simulink model "TrajectoryGenerator2DOF_freq"  (R2023b)
settings: Solver=FixedStepDiscrete  StartTime=0.0  StopTime=1.2*1.4  FixedStep=0.002  RelTol=1e-3
undefined symbols (not defined in the file or in its folder): M_z, Smoothers, Ts
(part 1 of 2)
settings Model: Creator=simon  LastModifiedBy=simon

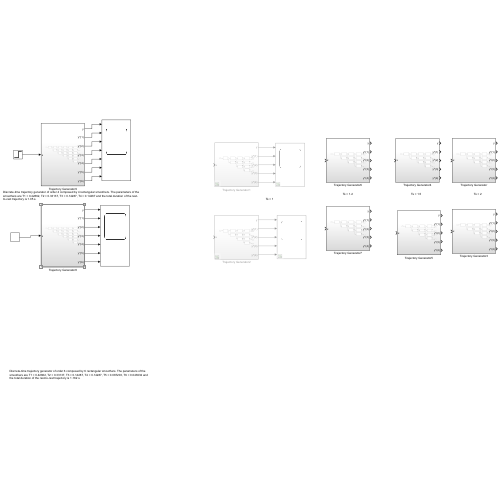
[thumbnail: Simulink's stored preview of the top-level diagram]
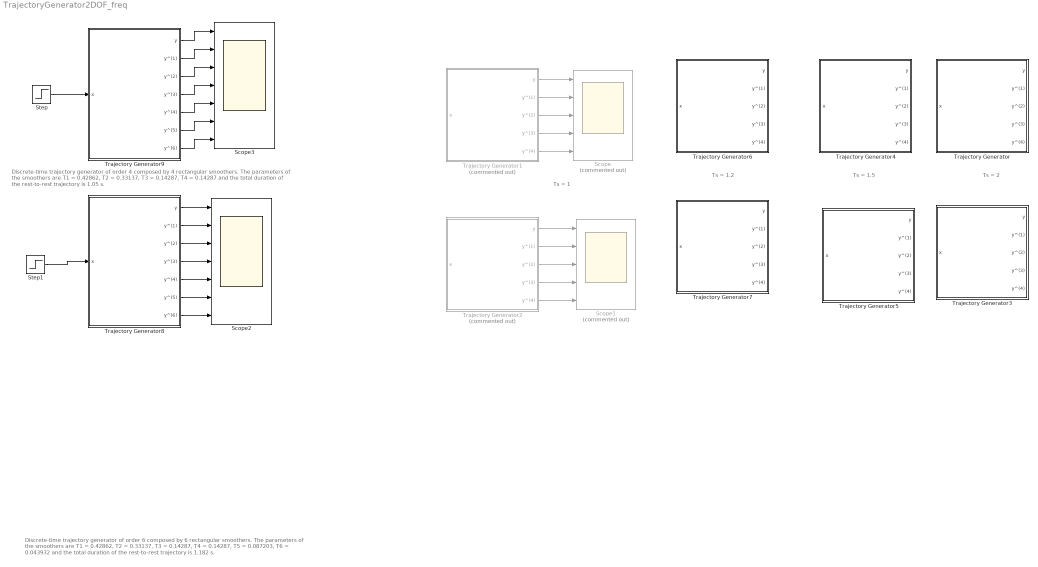
== system TrajectoryGenerator2DOF_freq ==
  note: Ts = 1
  note: Discrete-time trajectory generator of order 4 composed by 4 rectangular smoothers. The parameters of the smoothers are T1 = 0.42862, T2 = 0.33137, T3 = 0.14287, T4 = 0.14287 and the total duration of the rest-to-rest trajectory is 1.05 s.
  note: Ts = 2
  note: Ts = 1.5
  note: Ts = 1.2
  note: Discrete-time trajectory generator of order 6 composed by 6 rectangular smoothers. The parameters of the smoothers are T1 = 0.42862, T2 = 0.33137, T3 = 0.14287, T4 = 0.14287, T5 = 0.087203, T6 = 0.043932 and the total duration of the rest-to-rest trajectory is 1.182 s.
  Scope : Scope  Commented=on  NumInputPorts=5
  Scope1 : Scope  Commented=on  NumInputPorts=5
  Scope2 : Scope  NumInputPorts=7
  Scope3 : Scope  NumInputPorts=7
  Step : Step  Time=0  After=0.5  SampleTime=0.002
  Step1 : Step  Time=0.4*Ts  After=-0.5  SampleTime=0.002
  Trajectory Generator : Subsystem
  Trajectory Generator1 : Subsystem  Commented=on
  Trajectory Generator2 : Subsystem  Commented=on
  Trajectory Generator3 : Subsystem
  Trajectory Generator4 : Subsystem
  Trajectory Generator5 : Subsystem
  Trajectory Generator6 : Subsystem
  Trajectory Generator7 : Subsystem
  Trajectory Generator8 : Subsystem
  Trajectory Generator9 : Subsystem
  wires:
  Step/1 -> Trajectory Generator9/1(x)
  Step1/1 -> Trajectory Generator8/1(x)
  Trajectory Generator8/6(y^(5)) -> Scope2/6
  Trajectory Generator8/4(y^(3)) -> Scope2/4
  Trajectory Generator8/7(y^(6)) -> Scope2/7
  Trajectory Generator8/3(y^(2)) -> Scope2/3
  Trajectory Generator8/5(y^(4)) -> Scope2/5
  Trajectory Generator8/2(y^(1)) -> Scope2/2
  Trajectory Generator8/1(y) -> Scope2/1
  Trajectory Generator1/4(y^(3)) -> Scope/4
  Trajectory Generator1/5(y^(4)) -> Scope/5
  Trajectory Generator1/2(y^(1)) -> Scope/2
  Trajectory Generator1/1(y) -> Scope/1
  Trajectory Generator1/3(y^(2)) -> Scope/3
  Trajectory Generator9/5(y^(4)) -> Scope3/5
  Trajectory Generator9/1(y) -> Scope3/1
  Trajectory Generator9/2(y^(1)) -> Scope3/2
  Trajectory Generator9/4(y^(3)) -> Scope3/4
  Trajectory Generator9/3(y^(2)) -> Scope3/3
  Trajectory Generator9/6(y^(5)) -> Scope3/6
  Trajectory Generator9/7(y^(6)) -> Scope3/7
  Trajectory Generator2/2(y^(1)) -> Scope1/2
  Trajectory Generator2/3(y^(2)) -> Scope1/3
  Trajectory Generator2/4(y^(3)) -> Scope1/4
  Trajectory Generator2/5(y^(4)) -> Scope1/5
  Trajectory Generator2/1(y) -> Scope1/1

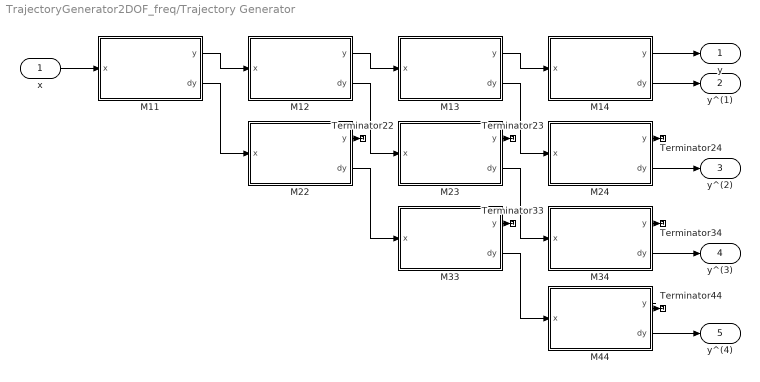
== system TrajectoryGenerator2DOF_freq/Trajectory Generator ==
  x : Inport
  M11 : Subsystem  AncestorBlock=Smoothers/M_z  mask{N=429, Ts=0.002, Q0=0}
      mask prompts: N "N_i"; Ts "Sampling period (Ts)"; Q0 "Initial position"
  M12 : Subsystem  AncestorBlock=Smoothers/M_z  mask{N=286, Ts=0.002, Q0=0}
      mask prompts: N "N_i"; Ts "Sampling period (Ts)"; Q0 "Initial position"
  M13 : Subsystem  AncestorBlock=Smoothers/M_z  mask{N=166, Ts=0.002, Q0=0}
      mask prompts: N "N_i"; Ts "Sampling period (Ts)"; Q0 "Initial position"
  M14 : Subsystem  AncestorBlock=Smoothers/M_z  mask{N=143, Ts=0.002, Q0=0}
      mask prompts: N "N_i"; Ts "Sampling period (Ts)"; Q0 "Initial position"
  M22 : Subsystem  AncestorBlock=Smoothers/M_z  mask{N=286, Ts=0.002, Q0=0}
      mask prompts: N "N_i"; Ts "Sampling period (Ts)"; Q0 "Initial position"
  M23 : Subsystem  AncestorBlock=Smoothers/M_z  mask{N=166, Ts=0.002, Q0=0}
      mask prompts: N "N_i"; Ts "Sampling period (Ts)"; Q0 "Initial position"
  M24 : Subsystem  AncestorBlock=Smoothers/M_z  mask{N=143, Ts=0.002, Q0=0}
      mask prompts: N "N_i"; Ts "Sampling period (Ts)"; Q0 "Initial position"
  M33 : Subsystem  AncestorBlock=Smoothers/M_z  mask{N=166, Ts=0.002, Q0=0}
      mask prompts: N "N_i"; Ts "Sampling period (Ts)"; Q0 "Initial position"
  M34 : Subsystem  AncestorBlock=Smoothers/M_z  mask{N=143, Ts=0.002, Q0=0}
      mask prompts: N "N_i"; Ts "Sampling period (Ts)"; Q0 "Initial position"
  M44 : Subsystem  AncestorBlock=Smoothers/M_z  mask{N=143, Ts=0.002, Q0=0}
      mask prompts: N "N_i"; Ts "Sampling period (Ts)"; Q0 "Initial position"
  Terminator{22..24,33..34,44} (6 alike) : Terminator
  y : Outport
  y^(1) : Outport  Port=2
  y^(2) : Outport  Port=3
  y^(3) : Outport  Port=4
  y^(4) : Outport  Port=5
  wires:
  x/1 -> M11/1(x)
  M11/1(y) -> M12/1(x)
  M12/1(y) -> M13/1(x)
  M13/1(y) -> M14/1(x)
  M11/2(dy) -> M22/1(x)
  M12/2(dy) -> M23/1(x)
  M13/2(dy) -> M24/1(x)
  M22/2(dy) -> M33/1(x)
  M23/2(dy) -> M34/1(x)
  M33/2(dy) -> M44/1(x)
  M22/1(y) -> Terminator22/1
  M23/1(y) -> Terminator23/1
  M24/1(y) -> Terminator24/1
  M33/1(y) -> Terminator33/1
  M34/1(y) -> Terminator34/1
  M44/1(y) -> Terminator44/1
  M14/1(y) -> y/1
  M14/2(dy) -> y^(1)/1
  M24/2(dy) -> y^(2)/1
  M34/2(dy) -> y^(3)/1
  M44/2(dy) -> y^(4)/1

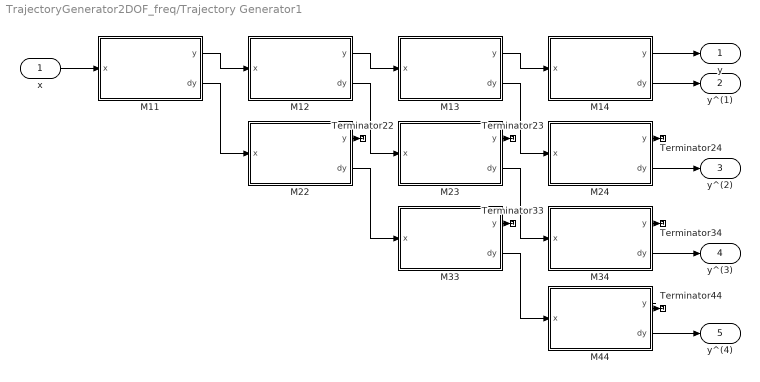
== system TrajectoryGenerator2DOF_freq/Trajectory Generator1 ==
  x : Inport
  M11 : Subsystem  AncestorBlock=Smoothers/M_z  mask{N=215, Ts=0.002, Q0=0}
      mask prompts: N "N_i"; Ts "Sampling period (Ts)"; Q0 "Initial position"
  M12 : Subsystem  AncestorBlock=Smoothers/M_z  mask{N=166, Ts=0.002, Q0=0}
      mask prompts: N "N_i"; Ts "Sampling period (Ts)"; Q0 "Initial position"
  M13 : Subsystem  AncestorBlock=Smoothers/M_z  mask{N=72, Ts=0.002, Q0=0}
      mask prompts: N "N_i"; Ts "Sampling period (Ts)"; Q0 "Initial position"
  M14 : Subsystem  AncestorBlock=Smoothers/M_z  mask{N=72, Ts=0.002, Q0=0}
      mask prompts: N "N_i"; Ts "Sampling period (Ts)"; Q0 "Initial position"
  M22 : Subsystem  AncestorBlock=Smoothers/M_z  mask{N=166, Ts=0.002, Q0=0}
      mask prompts: N "N_i"; Ts "Sampling period (Ts)"; Q0 "Initial position"
  M23 : Subsystem  AncestorBlock=Smoothers/M_z  mask{N=72, Ts=0.002, Q0=0}
      mask prompts: N "N_i"; Ts "Sampling period (Ts)"; Q0 "Initial position"
  M24 : Subsystem  AncestorBlock=Smoothers/M_z  mask{N=72, Ts=0.002, Q0=0}
      mask prompts: N "N_i"; Ts "Sampling period (Ts)"; Q0 "Initial position"
  M33 : Subsystem  AncestorBlock=Smoothers/M_z  mask{N=72, Ts=0.002, Q0=0}
      mask prompts: N "N_i"; Ts "Sampling period (Ts)"; Q0 "Initial position"
  M34 : Subsystem  AncestorBlock=Smoothers/M_z  mask{N=72, Ts=0.002, Q0=0}
      mask prompts: N "N_i"; Ts "Sampling period (Ts)"; Q0 "Initial position"
  M44 : Subsystem  AncestorBlock=Smoothers/M_z  mask{N=72, Ts=0.002, Q0=0}
      mask prompts: N "N_i"; Ts "Sampling period (Ts)"; Q0 "Initial position"
  Terminator{22..24,33..34,44} (6 alike) : Terminator
  y : Outport
  y^(1) : Outport  Port=2
  y^(2) : Outport  Port=3
  y^(3) : Outport  Port=4
  y^(4) : Outport  Port=5
  wires:
  x/1 -> M11/1(x)
  M11/1(y) -> M12/1(x)
  M12/1(y) -> M13/1(x)
  M13/1(y) -> M14/1(x)
  M11/2(dy) -> M22/1(x)
  M12/2(dy) -> M23/1(x)
  M13/2(dy) -> M24/1(x)
  M22/2(dy) -> M33/1(x)
  M23/2(dy) -> M34/1(x)
  M33/2(dy) -> M44/1(x)
  M22/1(y) -> Terminator22/1
  M23/1(y) -> Terminator23/1
  M24/1(y) -> Terminator24/1
  M33/1(y) -> Terminator33/1
  M34/1(y) -> Terminator34/1
  M44/1(y) -> Terminator44/1
  M14/1(y) -> y/1
  M14/2(dy) -> y^(1)/1
  M24/2(dy) -> y^(2)/1
  M34/2(dy) -> y^(3)/1
  M44/2(dy) -> y^(4)/1

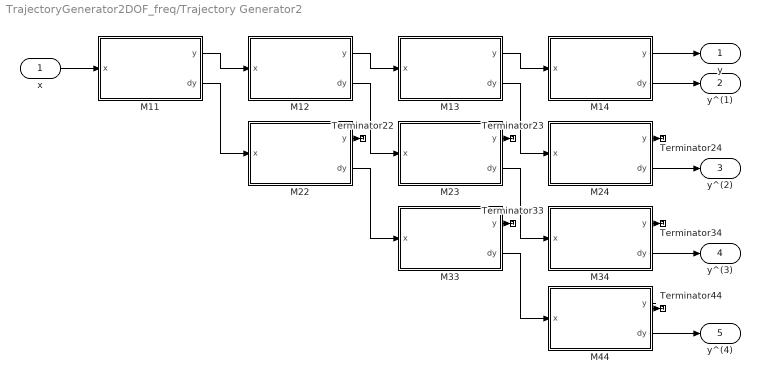
== system TrajectoryGenerator2DOF_freq/Trajectory Generator2 ==
  x : Inport
  M11 : Subsystem  AncestorBlock=Smoothers/M_z  mask{N=215, Ts=0.002, Q0=0}
      mask prompts: N "N_i"; Ts "Sampling period (Ts)"; Q0 "Initial position"
  M12 : Subsystem  AncestorBlock=Smoothers/M_z  mask{N=166, Ts=0.002, Q0=0}
      mask prompts: N "N_i"; Ts "Sampling period (Ts)"; Q0 "Initial position"
  M13 : Subsystem  AncestorBlock=Smoothers/M_z  mask{N=72, Ts=0.002, Q0=0}
      mask prompts: N "N_i"; Ts "Sampling period (Ts)"; Q0 "Initial position"
  M14 : Subsystem  AncestorBlock=Smoothers/M_z  mask{N=72, Ts=0.002, Q0=0}
      mask prompts: N "N_i"; Ts "Sampling period (Ts)"; Q0 "Initial position"
  M22 : Subsystem  AncestorBlock=Smoothers/M_z  mask{N=166, Ts=0.002, Q0=0}
      mask prompts: N "N_i"; Ts "Sampling period (Ts)"; Q0 "Initial position"
  M23 : Subsystem  AncestorBlock=Smoothers/M_z  mask{N=72, Ts=0.002, Q0=0}
      mask prompts: N "N_i"; Ts "Sampling period (Ts)"; Q0 "Initial position"
  M24 : Subsystem  AncestorBlock=Smoothers/M_z  mask{N=72, Ts=0.002, Q0=0}
      mask prompts: N "N_i"; Ts "Sampling period (Ts)"; Q0 "Initial position"
  M33 : Subsystem  AncestorBlock=Smoothers/M_z  mask{N=72, Ts=0.002, Q0=0}
      mask prompts: N "N_i"; Ts "Sampling period (Ts)"; Q0 "Initial position"
  M34 : Subsystem  AncestorBlock=Smoothers/M_z  mask{N=72, Ts=0.002, Q0=0}
      mask prompts: N "N_i"; Ts "Sampling period (Ts)"; Q0 "Initial position"
  M44 : Subsystem  AncestorBlock=Smoothers/M_z  mask{N=72, Ts=0.002, Q0=0}
      mask prompts: N "N_i"; Ts "Sampling period (Ts)"; Q0 "Initial position"
  Terminator{22..24,33..34,44} (6 alike) : Terminator
  y : Outport
  y^(1) : Outport  Port=2
  y^(2) : Outport  Port=3
  y^(3) : Outport  Port=4
  y^(4) : Outport  Port=5
  wires:
  x/1 -> M11/1(x)
  M11/1(y) -> M12/1(x)
  M12/1(y) -> M13/1(x)
  M13/1(y) -> M14/1(x)
  M11/2(dy) -> M22/1(x)
  M12/2(dy) -> M23/1(x)
  M13/2(dy) -> M24/1(x)
  M22/2(dy) -> M33/1(x)
  M23/2(dy) -> M34/1(x)
  M33/2(dy) -> M44/1(x)
  M22/1(y) -> Terminator22/1
  M23/1(y) -> Terminator23/1
  M24/1(y) -> Terminator24/1
  M33/1(y) -> Terminator33/1
  M34/1(y) -> Terminator34/1
  M44/1(y) -> Terminator44/1
  M14/1(y) -> y/1
  M14/2(dy) -> y^(1)/1
  M24/2(dy) -> y^(2)/1
  M34/2(dy) -> y^(3)/1
  M44/2(dy) -> y^(4)/1

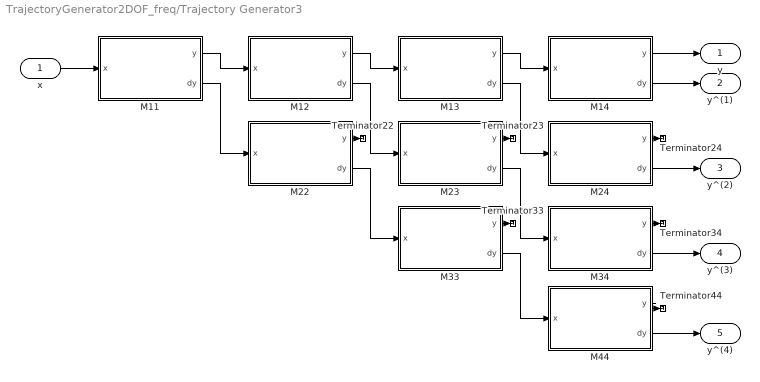
== system TrajectoryGenerator2DOF_freq/Trajectory Generator3 ==
  x : Inport
  M11 : Subsystem  AncestorBlock=Smoothers/M_z  mask{N=429, Ts=0.002, Q0=0}
      mask prompts: N "N_i"; Ts "Sampling period (Ts)"; Q0 "Initial position"
  M12 : Subsystem  AncestorBlock=Smoothers/M_z  mask{N=286, Ts=0.002, Q0=0}
      mask prompts: N "N_i"; Ts "Sampling period (Ts)"; Q0 "Initial position"
  M13 : Subsystem  AncestorBlock=Smoothers/M_z  mask{N=166, Ts=0.002, Q0=0}
      mask prompts: N "N_i"; Ts "Sampling period (Ts)"; Q0 "Initial position"
  M14 : Subsystem  AncestorBlock=Smoothers/M_z  mask{N=143, Ts=0.002, Q0=0}
      mask prompts: N "N_i"; Ts "Sampling period (Ts)"; Q0 "Initial position"
  M22 : Subsystem  AncestorBlock=Smoothers/M_z  mask{N=286, Ts=0.002, Q0=0}
      mask prompts: N "N_i"; Ts "Sampling period (Ts)"; Q0 "Initial position"
  M23 : Subsystem  AncestorBlock=Smoothers/M_z  mask{N=166, Ts=0.002, Q0=0}
      mask prompts: N "N_i"; Ts "Sampling period (Ts)"; Q0 "Initial position"
  M24 : Subsystem  AncestorBlock=Smoothers/M_z  mask{N=143, Ts=0.002, Q0=0}
      mask prompts: N "N_i"; Ts "Sampling period (Ts)"; Q0 "Initial position"
  M33 : Subsystem  AncestorBlock=Smoothers/M_z  mask{N=166, Ts=0.002, Q0=0}
      mask prompts: N "N_i"; Ts "Sampling period (Ts)"; Q0 "Initial position"
  M34 : Subsystem  AncestorBlock=Smoothers/M_z  mask{N=143, Ts=0.002, Q0=0}
      mask prompts: N "N_i"; Ts "Sampling period (Ts)"; Q0 "Initial position"
  M44 : Subsystem  AncestorBlock=Smoothers/M_z  mask{N=143, Ts=0.002, Q0=0}
      mask prompts: N "N_i"; Ts "Sampling period (Ts)"; Q0 "Initial position"
  Terminator{22..24,33..34,44} (6 alike) : Terminator
  y : Outport
  y^(1) : Outport  Port=2
  y^(2) : Outport  Port=3
  y^(3) : Outport  Port=4
  y^(4) : Outport  Port=5
  wires:
  x/1 -> M11/1(x)
  M11/1(y) -> M12/1(x)
  M12/1(y) -> M13/1(x)
  M13/1(y) -> M14/1(x)
  M11/2(dy) -> M22/1(x)
  M12/2(dy) -> M23/1(x)
  M13/2(dy) -> M24/1(x)
  M22/2(dy) -> M33/1(x)
  M23/2(dy) -> M34/1(x)
  M33/2(dy) -> M44/1(x)
  M22/1(y) -> Terminator22/1
  M23/1(y) -> Terminator23/1
  M24/1(y) -> Terminator24/1
  M33/1(y) -> Terminator33/1
  M34/1(y) -> Terminator34/1
  M44/1(y) -> Terminator44/1
  M14/1(y) -> y/1
  M14/2(dy) -> y^(1)/1
  M24/2(dy) -> y^(2)/1
  M34/2(dy) -> y^(3)/1
  M44/2(dy) -> y^(4)/1

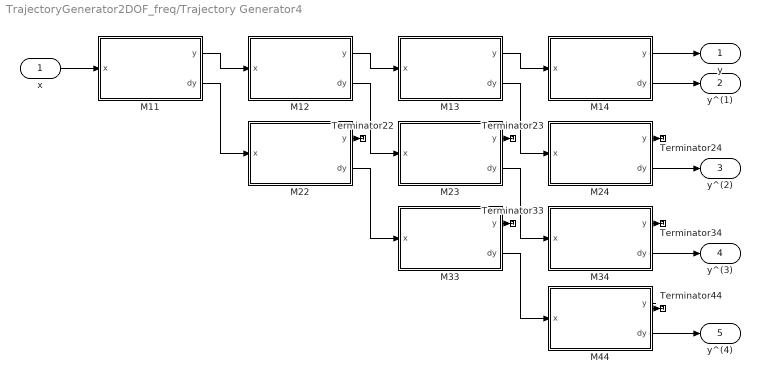
== system TrajectoryGenerator2DOF_freq/Trajectory Generator4 ==
  x : Inport
  M11 : Subsystem  AncestorBlock=Smoothers/M_z  mask{N=322, Ts=0.002, Q0=0}
      mask prompts: N "N_i"; Ts "Sampling period (Ts)"; Q0 "Initial position"
  M12 : Subsystem  AncestorBlock=Smoothers/M_z  mask{N=215, Ts=0.002, Q0=0}
      mask prompts: N "N_i"; Ts "Sampling period (Ts)"; Q0 "Initial position"
  M13 : Subsystem  AncestorBlock=Smoothers/M_z  mask{N=166, Ts=0.002, Q0=0}
      mask prompts: N "N_i"; Ts "Sampling period (Ts)"; Q0 "Initial position"
  M14 : Subsystem  AncestorBlock=Smoothers/M_z  mask{N=108, Ts=0.002, Q0=0}
      mask prompts: N "N_i"; Ts "Sampling period (Ts)"; Q0 "Initial position"
  M22 : Subsystem  AncestorBlock=Smoothers/M_z  mask{N=215, Ts=0.002, Q0=0}
      mask prompts: N "N_i"; Ts "Sampling period (Ts)"; Q0 "Initial position"
  M23 : Subsystem  AncestorBlock=Smoothers/M_z  mask{N=166, Ts=0.002, Q0=0}
      mask prompts: N "N_i"; Ts "Sampling period (Ts)"; Q0 "Initial position"
  M24 : Subsystem  AncestorBlock=Smoothers/M_z  mask{N=108, Ts=0.002, Q0=0}
      mask prompts: N "N_i"; Ts "Sampling period (Ts)"; Q0 "Initial position"
  M33 : Subsystem  AncestorBlock=Smoothers/M_z  mask{N=166, Ts=0.002, Q0=0}
      mask prompts: N "N_i"; Ts "Sampling period (Ts)"; Q0 "Initial position"
  M34 : Subsystem  AncestorBlock=Smoothers/M_z  mask{N=108, Ts=0.002, Q0=0}
      mask prompts: N "N_i"; Ts "Sampling period (Ts)"; Q0 "Initial position"
  M44 : Subsystem  AncestorBlock=Smoothers/M_z  mask{N=108, Ts=0.002, Q0=0}
      mask prompts: N "N_i"; Ts "Sampling period (Ts)"; Q0 "Initial position"
  Terminator{22..24,33..34,44} (6 alike) : Terminator
  y : Outport
  y^(1) : Outport  Port=2
  y^(2) : Outport  Port=3
  y^(3) : Outport  Port=4
  y^(4) : Outport  Port=5
  wires:
  x/1 -> M11/1(x)
  M11/1(y) -> M12/1(x)
  M12/1(y) -> M13/1(x)
  M13/1(y) -> M14/1(x)
  M11/2(dy) -> M22/1(x)
  M12/2(dy) -> M23/1(x)
  M13/2(dy) -> M24/1(x)
  M22/2(dy) -> M33/1(x)
  M23/2(dy) -> M34/1(x)
  M33/2(dy) -> M44/1(x)
  M22/1(y) -> Terminator22/1
  M23/1(y) -> Terminator23/1
  M24/1(y) -> Terminator24/1
  M33/1(y) -> Terminator33/1
  M34/1(y) -> Terminator34/1
  M44/1(y) -> Terminator44/1
  M14/1(y) -> y/1
  M14/2(dy) -> y^(1)/1
  M24/2(dy) -> y^(2)/1
  M34/2(dy) -> y^(3)/1
  M44/2(dy) -> y^(4)/1

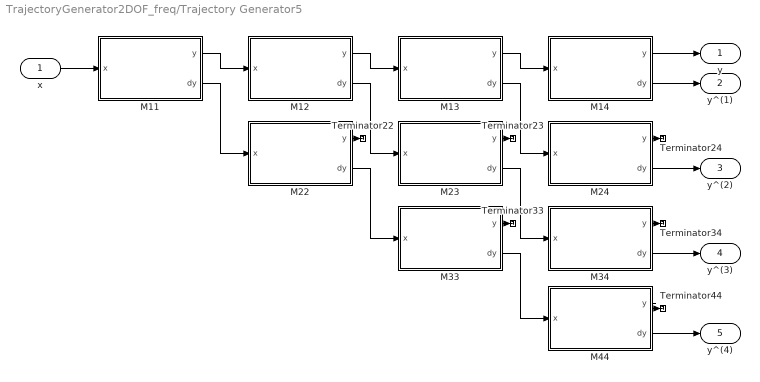
== system TrajectoryGenerator2DOF_freq/Trajectory Generator5 ==
  x : Inport
  M11 : Subsystem  AncestorBlock=Smoothers/M_z  mask{N=322, Ts=0.002, Q0=0}
      mask prompts: N "N_i"; Ts "Sampling period (Ts)"; Q0 "Initial position"
  M12 : Subsystem  AncestorBlock=Smoothers/M_z  mask{N=215, Ts=0.002, Q0=0}
      mask prompts: N "N_i"; Ts "Sampling period (Ts)"; Q0 "Initial position"
  M13 : Subsystem  AncestorBlock=Smoothers/M_z  mask{N=166, Ts=0.002, Q0=0}
      mask prompts: N "N_i"; Ts "Sampling period (Ts)"; Q0 "Initial position"
  M14 : Subsystem  AncestorBlock=Smoothers/M_z  mask{N=108, Ts=0.002, Q0=0}
      mask prompts: N "N_i"; Ts "Sampling period (Ts)"; Q0 "Initial position"
  M22 : Subsystem  AncestorBlock=Smoothers/M_z  mask{N=215, Ts=0.002, Q0=0}
      mask prompts: N "N_i"; Ts "Sampling period (Ts)"; Q0 "Initial position"
  M23 : Subsystem  AncestorBlock=Smoothers/M_z  mask{N=166, Ts=0.002, Q0=0}
      mask prompts: N "N_i"; Ts "Sampling period (Ts)"; Q0 "Initial position"
  M24 : Subsystem  AncestorBlock=Smoothers/M_z  mask{N=108, Ts=0.002, Q0=0}
      mask prompts: N "N_i"; Ts "Sampling period (Ts)"; Q0 "Initial position"
  M33 : Subsystem  AncestorBlock=Smoothers/M_z  mask{N=166, Ts=0.002, Q0=0}
      mask prompts: N "N_i"; Ts "Sampling period (Ts)"; Q0 "Initial position"
  M34 : Subsystem  AncestorBlock=Smoothers/M_z  mask{N=108, Ts=0.002, Q0=0}
      mask prompts: N "N_i"; Ts "Sampling period (Ts)"; Q0 "Initial position"
  M44 : Subsystem  AncestorBlock=Smoothers/M_z  mask{N=108, Ts=0.002, Q0=0}
      mask prompts: N "N_i"; Ts "Sampling period (Ts)"; Q0 "Initial position"
  Terminator{22..24,33..34,44} (6 alike) : Terminator
  y : Outport
  y^(1) : Outport  Port=2
  y^(2) : Outport  Port=3
  y^(3) : Outport  Port=4
  y^(4) : Outport  Port=5
  wires:
  x/1 -> M11/1(x)
  M11/1(y) -> M12/1(x)
  M12/1(y) -> M13/1(x)
  M13/1(y) -> M14/1(x)
  M11/2(dy) -> M22/1(x)
  M12/2(dy) -> M23/1(x)
  M13/2(dy) -> M24/1(x)
  M22/2(dy) -> M33/1(x)
  M23/2(dy) -> M34/1(x)
  M33/2(dy) -> M44/1(x)
  M22/1(y) -> Terminator22/1
  M23/1(y) -> Terminator23/1
  M24/1(y) -> Terminator24/1
  M33/1(y) -> Terminator33/1
  M34/1(y) -> Terminator34/1
  M44/1(y) -> Terminator44/1
  M14/1(y) -> y/1
  M14/2(dy) -> y^(1)/1
  M24/2(dy) -> y^(2)/1
  M34/2(dy) -> y^(3)/1
  M44/2(dy) -> y^(4)/1

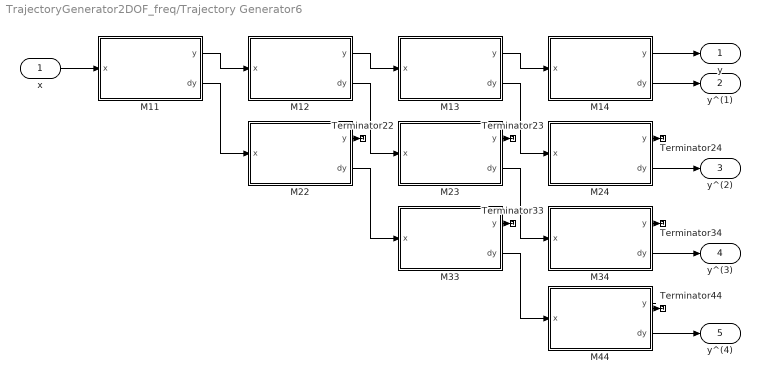
== system TrajectoryGenerator2DOF_freq/Trajectory Generator6 ==
  x : Inport
  M11 : Subsystem  AncestorBlock=Smoothers/M_z  mask{N=258, Ts=0.002, Q0=0}
      mask prompts: N "N_i"; Ts "Sampling period (Ts)"; Q0 "Initial position"
  M12 : Subsystem  AncestorBlock=Smoothers/M_z  mask{N=172, Ts=0.002, Q0=0}
      mask prompts: N "N_i"; Ts "Sampling period (Ts)"; Q0 "Initial position"
  M13 : Subsystem  AncestorBlock=Smoothers/M_z  mask{N=166, Ts=0.002, Q0=0}
      mask prompts: N "N_i"; Ts "Sampling period (Ts)"; Q0 "Initial position"
  M14 : Subsystem  AncestorBlock=Smoothers/M_z  mask{N=86, Ts=0.002, Q0=0}
      mask prompts: N "N_i"; Ts "Sampling period (Ts)"; Q0 "Initial position"
  M22 : Subsystem  AncestorBlock=Smoothers/M_z  mask{N=172, Ts=0.002, Q0=0}
      mask prompts: N "N_i"; Ts "Sampling period (Ts)"; Q0 "Initial position"
  M23 : Subsystem  AncestorBlock=Smoothers/M_z  mask{N=166, Ts=0.002, Q0=0}
      mask prompts: N "N_i"; Ts "Sampling period (Ts)"; Q0 "Initial position"
  M24 : Subsystem  AncestorBlock=Smoothers/M_z  mask{N=86, Ts=0.002, Q0=0}
      mask prompts: N "N_i"; Ts "Sampling period (Ts)"; Q0 "Initial position"
  M33 : Subsystem  AncestorBlock=Smoothers/M_z  mask{N=166, Ts=0.002, Q0=0}
      mask prompts: N "N_i"; Ts "Sampling period (Ts)"; Q0 "Initial position"
  M34 : Subsystem  AncestorBlock=Smoothers/M_z  mask{N=86, Ts=0.002, Q0=0}
      mask prompts: N "N_i"; Ts "Sampling period (Ts)"; Q0 "Initial position"
  M44 : Subsystem  AncestorBlock=Smoothers/M_z  mask{N=86, Ts=0.002, Q0=0}
      mask prompts: N "N_i"; Ts "Sampling period (Ts)"; Q0 "Initial position"
  Terminator{22..24,33..34,44} (6 alike) : Terminator
  y : Outport
  y^(1) : Outport  Port=2
  y^(2) : Outport  Port=3
  y^(3) : Outport  Port=4
  y^(4) : Outport  Port=5
  wires:
  x/1 -> M11/1(x)
  M11/1(y) -> M12/1(x)
  M12/1(y) -> M13/1(x)
  M13/1(y) -> M14/1(x)
  M11/2(dy) -> M22/1(x)
  M12/2(dy) -> M23/1(x)
  M13/2(dy) -> M24/1(x)
  M22/2(dy) -> M33/1(x)
  M23/2(dy) -> M34/1(x)
  M33/2(dy) -> M44/1(x)
  M22/1(y) -> Terminator22/1
  M23/1(y) -> Terminator23/1
  M24/1(y) -> Terminator24/1
  M33/1(y) -> Terminator33/1
  M34/1(y) -> Terminator34/1
  M44/1(y) -> Terminator44/1
  M14/1(y) -> y/1
  M14/2(dy) -> y^(1)/1
  M24/2(dy) -> y^(2)/1
  M34/2(dy) -> y^(3)/1
  M44/2(dy) -> y^(4)/1

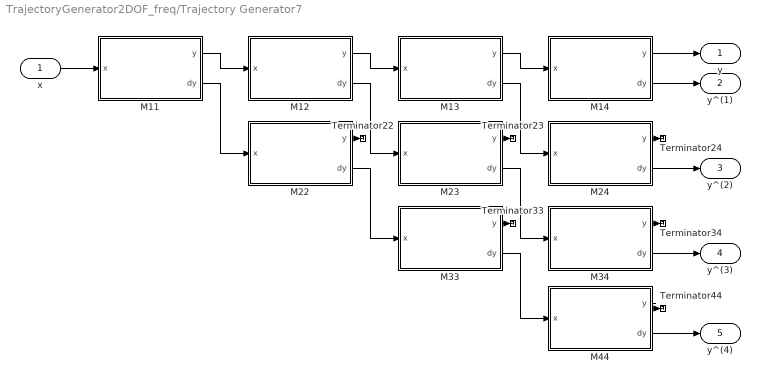
== system TrajectoryGenerator2DOF_freq/Trajectory Generator7 ==
  x : Inport
  M11 : Subsystem  AncestorBlock=Smoothers/M_z  mask{N=258, Ts=0.002, Q0=0}
      mask prompts: N "N_i"; Ts "Sampling period (Ts)"; Q0 "Initial position"
  M12 : Subsystem  AncestorBlock=Smoothers/M_z  mask{N=172, Ts=0.002, Q0=0}
      mask prompts: N "N_i"; Ts "Sampling period (Ts)"; Q0 "Initial position"
  M13 : Subsystem  AncestorBlock=Smoothers/M_z  mask{N=166, Ts=0.002, Q0=0}
      mask prompts: N "N_i"; Ts "Sampling period (Ts)"; Q0 "Initial position"
  M14 : Subsystem  AncestorBlock=Smoothers/M_z  mask{N=86, Ts=0.002, Q0=0}
      mask prompts: N "N_i"; Ts "Sampling period (Ts)"; Q0 "Initial position"
  M22 : Subsystem  AncestorBlock=Smoothers/M_z  mask{N=172, Ts=0.002, Q0=0}
      mask prompts: N "N_i"; Ts "Sampling period (Ts)"; Q0 "Initial position"
  M23 : Subsystem  AncestorBlock=Smoothers/M_z  mask{N=166, Ts=0.002, Q0=0}
      mask prompts: N "N_i"; Ts "Sampling period (Ts)"; Q0 "Initial position"
  M24 : Subsystem  AncestorBlock=Smoothers/M_z  mask{N=86, Ts=0.002, Q0=0}
      mask prompts: N "N_i"; Ts "Sampling period (Ts)"; Q0 "Initial position"
  M33 : Subsystem  AncestorBlock=Smoothers/M_z  mask{N=166, Ts=0.002, Q0=0}
      mask prompts: N "N_i"; Ts "Sampling period (Ts)"; Q0 "Initial position"
  M34 : Subsystem  AncestorBlock=Smoothers/M_z  mask{N=86, Ts=0.002, Q0=0}
      mask prompts: N "N_i"; Ts "Sampling period (Ts)"; Q0 "Initial position"
  M44 : Subsystem  AncestorBlock=Smoothers/M_z  mask{N=86, Ts=0.002, Q0=0}
      mask prompts: N "N_i"; Ts "Sampling period (Ts)"; Q0 "Initial position"
  Terminator{22..24,33..34,44} (6 alike) : Terminator
  y : Outport
  y^(1) : Outport  Port=2
  y^(2) : Outport  Port=3
  y^(3) : Outport  Port=4
  y^(4) : Outport  Port=5
  wires:
  x/1 -> M11/1(x)
  M11/1(y) -> M12/1(x)
  M12/1(y) -> M13/1(x)
  M13/1(y) -> M14/1(x)
  M11/2(dy) -> M22/1(x)
  M12/2(dy) -> M23/1(x)
  M13/2(dy) -> M24/1(x)
  M22/2(dy) -> M33/1(x)
  M23/2(dy) -> M34/1(x)
  M33/2(dy) -> M44/1(x)
  M22/1(y) -> Terminator22/1
  M23/1(y) -> Terminator23/1
  M24/1(y) -> Terminator24/1
  M33/1(y) -> Terminator33/1
  M34/1(y) -> Terminator34/1
  M44/1(y) -> Terminator44/1
  M14/1(y) -> y/1
  M14/2(dy) -> y^(1)/1
  M24/2(dy) -> y^(2)/1
  M34/2(dy) -> y^(3)/1
  M44/2(dy) -> y^(4)/1

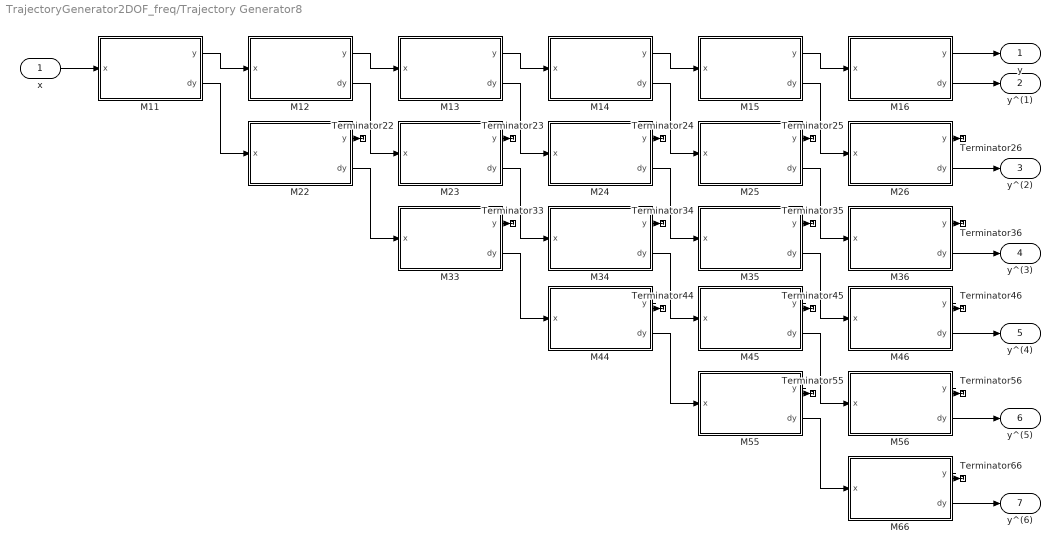
== system TrajectoryGenerator2DOF_freq/Trajectory Generator8 ==
  x : Inport
  M11 : Subsystem  AncestorBlock=Smoothers/M_z  mask{N=215, Ts=0.002, Q0=0}
      mask prompts: N "N_i"; Ts "Sampling period (Ts)"; Q0 "Initial position"
  M12 : Subsystem  AncestorBlock=Smoothers/M_z  mask{N=166, Ts=0.002, Q0=0}
      mask prompts: N "N_i"; Ts "Sampling period (Ts)"; Q0 "Initial position"
  M13 : Subsystem  AncestorBlock=Smoothers/M_z  mask{N=72, Ts=0.002, Q0=0}
      mask prompts: N "N_i"; Ts "Sampling period (Ts)"; Q0 "Initial position"
  M14 : Subsystem  AncestorBlock=Smoothers/M_z  mask{N=72, Ts=0.002, Q0=0}
      mask prompts: N "N_i"; Ts "Sampling period (Ts)"; Q0 "Initial position"
  M15 : Subsystem  AncestorBlock=Smoothers/M_z  mask{N=44, Ts=0.002, Q0=0}
      mask prompts: N "N_i"; Ts "Sampling period (Ts)"; Q0 "Initial position"
  M16 : Subsystem  AncestorBlock=Smoothers/M_z  mask{N=22, Ts=0.002, Q0=0}
      mask prompts: N "N_i"; Ts "Sampling period (Ts)"; Q0 "Initial position"
  M22 : Subsystem  AncestorBlock=Smoothers/M_z  mask{N=166, Ts=0.002, Q0=0}
      mask prompts: N "N_i"; Ts "Sampling period (Ts)"; Q0 "Initial position"
  M23 : Subsystem  AncestorBlock=Smoothers/M_z  mask{N=72, Ts=0.002, Q0=0}
      mask prompts: N "N_i"; Ts "Sampling period (Ts)"; Q0 "Initial position"
  M24 : Subsystem  AncestorBlock=Smoothers/M_z  mask{N=72, Ts=0.002, Q0=0}
      mask prompts: N "N_i"; Ts "Sampling period (Ts)"; Q0 "Initial position"
  M25 : Subsystem  AncestorBlock=Smoothers/M_z  mask{N=44, Ts=0.002, Q0=0}
      mask prompts: N "N_i"; Ts "Sampling period (Ts)"; Q0 "Initial position"
  M26 : Subsystem  AncestorBlock=Smoothers/M_z  mask{N=22, Ts=0.002, Q0=0}
      mask prompts: N "N_i"; Ts "Sampling period (Ts)"; Q0 "Initial position"
  M33 : Subsystem  AncestorBlock=Smoothers/M_z  mask{N=72, Ts=0.002, Q0=0}
      mask prompts: N "N_i"; Ts "Sampling period (Ts)"; Q0 "Initial position"
  M34 : Subsystem  AncestorBlock=Smoothers/M_z  mask{N=72, Ts=0.002, Q0=0}
      mask prompts: N "N_i"; Ts "Sampling period (Ts)"; Q0 "Initial position"
  M35 : Subsystem  AncestorBlock=Smoothers/M_z  mask{N=44, Ts=0.002, Q0=0}
      mask prompts: N "N_i"; Ts "Sampling period (Ts)"; Q0 "Initial position"
  M36 : Subsystem  AncestorBlock=Smoothers/M_z  mask{N=22, Ts=0.002, Q0=0}
      mask prompts: N "N_i"; Ts "Sampling period (Ts)"; Q0 "Initial position"
  M44 : Subsystem  AncestorBlock=Smoothers/M_z  mask{N=72, Ts=0.002, Q0=0}
      mask prompts: N "N_i"; Ts "Sampling period (Ts)"; Q0 "Initial position"
  M45 : Subsystem  AncestorBlock=Smoothers/M_z  mask{N=44, Ts=0.002, Q0=0}
      mask prompts: N "N_i"; Ts "Sampling period (Ts)"; Q0 "Initial position"
  M46 : Subsystem  AncestorBlock=Smoothers/M_z  mask{N=22, Ts=0.002, Q0=0}
      mask prompts: N "N_i"; Ts "Sampling period (Ts)"; Q0 "Initial position"
  M55 : Subsystem  AncestorBlock=Smoothers/M_z  mask{N=44, Ts=0.002, Q0=0}
      mask prompts: N "N_i"; Ts "Sampling period (Ts)"; Q0 "Initial position"
  M56 : Subsystem  AncestorBlock=Smoothers/M_z  mask{N=22, Ts=0.002, Q0=0}
      mask prompts: N "N_i"; Ts "Sampling period (Ts)"; Q0 "Initial position"
  M66 : Subsystem  AncestorBlock=Smoothers/M_z  mask{N=22, Ts=0.002, Q0=0}
      mask prompts: N "N_i"; Ts "Sampling period (Ts)"; Q0 "Initial position"
  Terminator{22..26,33..36,44..46,55..56,66} (15 alike) : Terminator
  y : Outport
  y^(1) : Outport  Port=2
  y^(2) : Outport  Port=3
  y^(3) : Outport  Port=4
  y^(4) : Outport  Port=5
  y^(5) : Outport  Port=6
  y^(6) : Outport  Port=7
  wires:
  x/1 -> M11/1(x)
  M11/1(y) -> M12/1(x)
  M12/1(y) -> M13/1(x)
  M13/1(y) -> M14/1(x)
  M14/1(y) -> M15/1(x)
  M15/1(y) -> M16/1(x)
  M11/2(dy) -> M22/1(x)
  M12/2(dy) -> M23/1(x)
  M13/2(dy) -> M24/1(x)
  M14/2(dy) -> M25/1(x)
  M15/2(dy) -> M26/1(x)
  M22/2(dy) -> M33/1(x)
  M23/2(dy) -> M34/1(x)
  M24/2(dy) -> M35/1(x)
  M25/2(dy) -> M36/1(x)
  M33/2(dy) -> M44/1(x)
  M34/2(dy) -> M45/1(x)
  M35/2(dy) -> M46/1(x)
  M44/2(dy) -> M55/1(x)
  M45/2(dy) -> M56/1(x)
  M55/2(dy) -> M66/1(x)
  M22/1(y) -> Terminator22/1
  M23/1(y) -> Terminator23/1
  M24/1(y) -> Terminator24/1
  M25/1(y) -> Terminator25/1
  M26/1(y) -> Terminator26/1
  M33/1(y) -> Terminator33/1
  M34/1(y) -> Terminator34/1
  M35/1(y) -> Terminator35/1
  M36/1(y) -> Terminator36/1
  M44/1(y) -> Terminator44/1
  M45/1(y) -> Terminator45/1
  M46/1(y) -> Terminator46/1
  M55/1(y) -> Terminator55/1
  M56/1(y) -> Terminator56/1
  M66/1(y) -> Terminator66/1
  M16/1(y) -> y/1
  M16/2(dy) -> y^(1)/1
  M26/2(dy) -> y^(2)/1
  M36/2(dy) -> y^(3)/1
  M46/2(dy) -> y^(4)/1
  M56/2(dy) -> y^(5)/1
  M66/2(dy) -> y^(6)/1

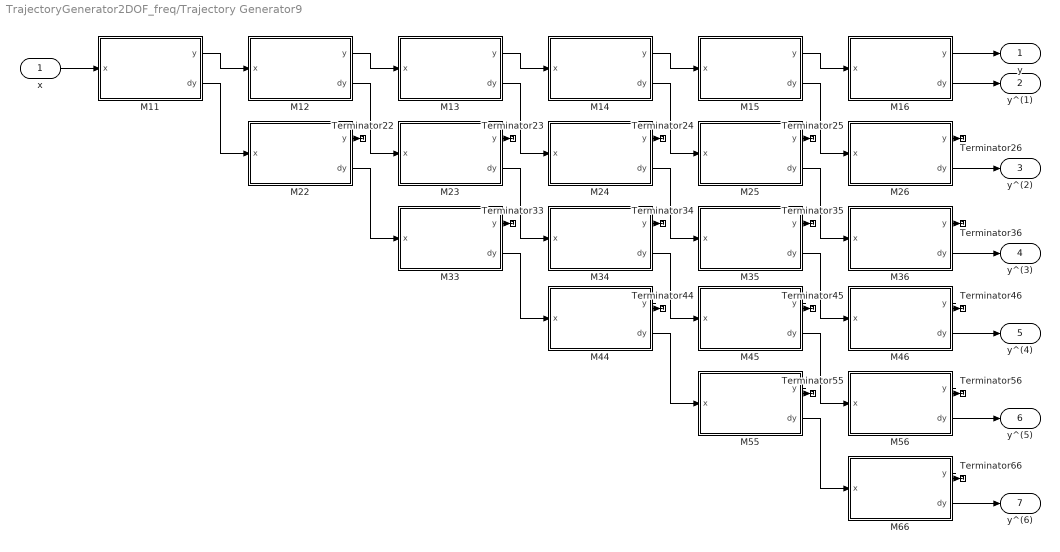
== system TrajectoryGenerator2DOF_freq/Trajectory Generator9 ==
  x : Inport
  M11 : Subsystem  AncestorBlock=Smoothers/M_z  mask{N=215, Ts=0.002, Q0=0}
      mask prompts: N "N_i"; Ts "Sampling period (Ts)"; Q0 "Initial position"
  M12 : Subsystem  AncestorBlock=Smoothers/M_z  mask{N=166, Ts=0.002, Q0=0}
      mask prompts: N "N_i"; Ts "Sampling period (Ts)"; Q0 "Initial position"
  M13 : Subsystem  AncestorBlock=Smoothers/M_z  mask{N=72, Ts=0.002, Q0=0}
      mask prompts: N "N_i"; Ts "Sampling period (Ts)"; Q0 "Initial position"
  M14 : Subsystem  AncestorBlock=Smoothers/M_z  mask{N=72, Ts=0.002, Q0=0}
      mask prompts: N "N_i"; Ts "Sampling period (Ts)"; Q0 "Initial position"
  M15 : Subsystem  AncestorBlock=Smoothers/M_z  mask{N=44, Ts=0.002, Q0=0}
      mask prompts: N "N_i"; Ts "Sampling period (Ts)"; Q0 "Initial position"
  M16 : Subsystem  AncestorBlock=Smoothers/M_z  mask{N=22, Ts=0.002, Q0=0}
      mask prompts: N "N_i"; Ts "Sampling period (Ts)"; Q0 "Initial position"
  M22 : Subsystem  AncestorBlock=Smoothers/M_z  mask{N=166, Ts=0.002, Q0=0}
      mask prompts: N "N_i"; Ts "Sampling period (Ts)"; Q0 "Initial position"
  M23 : Subsystem  AncestorBlock=Smoothers/M_z  mask{N=72, Ts=0.002, Q0=0}
      mask prompts: N "N_i"; Ts "Sampling period (Ts)"; Q0 "Initial position"
  M24 : Subsystem  AncestorBlock=Smoothers/M_z  mask{N=72, Ts=0.002, Q0=0}
      mask prompts: N "N_i"; Ts "Sampling period (Ts)"; Q0 "Initial position"
  M25 : Subsystem  AncestorBlock=Smoothers/M_z  mask{N=44, Ts=0.002, Q0=0}
      mask prompts: N "N_i"; Ts "Sampling period (Ts)"; Q0 "Initial position"
  M26 : Subsystem  AncestorBlock=Smoothers/M_z  mask{N=22, Ts=0.002, Q0=0}
      mask prompts: N "N_i"; Ts "Sampling period (Ts)"; Q0 "Initial position"
  M33 : Subsystem  AncestorBlock=Smoothers/M_z  mask{N=72, Ts=0.002, Q0=0}
      mask prompts: N "N_i"; Ts "Sampling period (Ts)"; Q0 "Initial position"
  M34 : Subsystem  AncestorBlock=Smoothers/M_z  mask{N=72, Ts=0.002, Q0=0}
      mask prompts: N "N_i"; Ts "Sampling period (Ts)"; Q0 "Initial position"
  M35 : Subsystem  AncestorBlock=Smoothers/M_z  mask{N=44, Ts=0.002, Q0=0}
      mask prompts: N "N_i"; Ts "Sampling period (Ts)"; Q0 "Initial position"
  M36 : Subsystem  AncestorBlock=Smoothers/M_z  mask{N=22, Ts=0.002, Q0=0}
      mask prompts: N "N_i"; Ts "Sampling period (Ts)"; Q0 "Initial position"
  M44 : Subsystem  AncestorBlock=Smoothers/M_z  mask{N=72, Ts=0.002, Q0=0}
      mask prompts: N "N_i"; Ts "Sampling period (Ts)"; Q0 "Initial position"
  M45 : Subsystem  AncestorBlock=Smoothers/M_z  mask{N=44, Ts=0.002, Q0=0}
      mask prompts: N "N_i"; Ts "Sampling period (Ts)"; Q0 "Initial position"
  M46 : Subsystem  AncestorBlock=Smoothers/M_z  mask{N=22, Ts=0.002, Q0=0}
      mask prompts: N "N_i"; Ts "Sampling period (Ts)"; Q0 "Initial position"
  M55 : Subsystem  AncestorBlock=Smoothers/M_z  mask{N=44, Ts=0.002, Q0=0}
      mask prompts: N "N_i"; Ts "Sampling period (Ts)"; Q0 "Initial position"
  M56 : Subsystem  AncestorBlock=Smoothers/M_z  mask{N=22, Ts=0.002, Q0=0}
      mask prompts: N "N_i"; Ts "Sampling period (Ts)"; Q0 "Initial position"
  M66 : Subsystem  AncestorBlock=Smoothers/M_z  mask{N=22, Ts=0.002, Q0=0}
      mask prompts: N "N_i"; Ts "Sampling period (Ts)"; Q0 "Initial position"
  Terminator{22..26,33..36,44..46,55..56,66} (15 alike) : Terminator
  y : Outport
  y^(1) : Outport  Port=2
  y^(2) : Outport  Port=3
  y^(3) : Outport  Port=4
  y^(4) : Outport  Port=5
  y^(5) : Outport  Port=6
  y^(6) : Outport  Port=7
  wires:
  x/1 -> M11/1(x)
  M11/1(y) -> M12/1(x)
  M12/1(y) -> M13/1(x)
  M13/1(y) -> M14/1(x)
  M14/1(y) -> M15/1(x)
  M15/1(y) -> M16/1(x)
  M11/2(dy) -> M22/1(x)
  M12/2(dy) -> M23/1(x)
  M13/2(dy) -> M24/1(x)
  M14/2(dy) -> M25/1(x)
  M15/2(dy) -> M26/1(x)
  M22/2(dy) -> M33/1(x)
  M23/2(dy) -> M34/1(x)
  M24/2(dy) -> M35/1(x)
  M25/2(dy) -> M36/1(x)
  M33/2(dy) -> M44/1(x)
  M34/2(dy) -> M45/1(x)
  M35/2(dy) -> M46/1(x)
  M44/2(dy) -> M55/1(x)
  M45/2(dy) -> M56/1(x)
  M55/2(dy) -> M66/1(x)
  M22/1(y) -> Terminator22/1
  M23/1(y) -> Terminator23/1
  M24/1(y) -> Terminator24/1
  M25/1(y) -> Terminator25/1
  M26/1(y) -> Terminator26/1
  M33/1(y) -> Terminator33/1
  M34/1(y) -> Terminator34/1
  M35/1(y) -> Terminator35/1
  M36/1(y) -> Terminator36/1
  M44/1(y) -> Terminator44/1
  M45/1(y) -> Terminator45/1
  M46/1(y) -> Terminator46/1
  M55/1(y) -> Terminator55/1
  M56/1(y) -> Terminator56/1
  M66/1(y) -> Terminator66/1
  M16/1(y) -> y/1
  M16/2(dy) -> y^(1)/1
  M26/2(dy) -> y^(2)/1
  M36/2(dy) -> y^(3)/1
  M46/2(dy) -> y^(4)/1
  M56/2(dy) -> y^(5)/1
  M66/2(dy) -> y^(6)/1

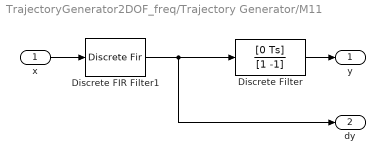
== system TrajectoryGenerator2DOF_freq/Trajectory Generator/M11 ==
  x : Inport
  Discrete FIR Filter1 : DiscreteFir  Coefficients=1/N/Ts*[1 zeros(1,N-1) -1]  InitialStates=Q0  SampleTime=Ts
  Discrete Filter : DiscreteFilter  Numerator=[0 Ts]  Denominator=[1 -1]  InitialStates=Q0  SampleTime=Ts
  y : Outport
  dy : Outport  Port=2
  wires:
  Discrete FIR Filter1/1 -> Discrete Filter/1, dy/1
  x/1 -> Discrete FIR Filter1/1
  Discrete Filter/1 -> y/1

== system TrajectoryGenerator2DOF_freq/Trajectory Generator/M12 ==
  x : Inport
  Discrete FIR Filter1 : DiscreteFir  Coefficients=1/N/Ts*[1 zeros(1,N-1) -1]  InitialStates=Q0  SampleTime=Ts
  Discrete Filter : DiscreteFilter  Numerator=[0 Ts]  Denominator=[1 -1]  InitialStates=Q0  SampleTime=Ts
  y : Outport
  dy : Outport  Port=2
  wires:
  Discrete FIR Filter1/1 -> Discrete Filter/1, dy/1
  x/1 -> Discrete FIR Filter1/1
  Discrete Filter/1 -> y/1

== system TrajectoryGenerator2DOF_freq/Trajectory Generator/M13 ==
  x : Inport
  Discrete FIR Filter1 : DiscreteFir  Coefficients=1/N/Ts*[1 zeros(1,N-1) -1]  InitialStates=Q0  SampleTime=Ts
  Discrete Filter : DiscreteFilter  Numerator=[0 Ts]  Denominator=[1 -1]  InitialStates=Q0  SampleTime=Ts
  y : Outport
  dy : Outport  Port=2
  wires:
  Discrete FIR Filter1/1 -> Discrete Filter/1, dy/1
  x/1 -> Discrete FIR Filter1/1
  Discrete Filter/1 -> y/1

== system TrajectoryGenerator2DOF_freq/Trajectory Generator/M14 ==
  x : Inport
  Discrete FIR Filter1 : DiscreteFir  Coefficients=1/N/Ts*[1 zeros(1,N-1) -1]  InitialStates=Q0  SampleTime=Ts
  Discrete Filter : DiscreteFilter  Numerator=[0 Ts]  Denominator=[1 -1]  InitialStates=Q0  SampleTime=Ts
  y : Outport
  dy : Outport  Port=2
  wires:
  Discrete FIR Filter1/1 -> Discrete Filter/1, dy/1
  x/1 -> Discrete FIR Filter1/1
  Discrete Filter/1 -> y/1

== system TrajectoryGenerator2DOF_freq/Trajectory Generator/M22 ==
  x : Inport
  Discrete FIR Filter1 : DiscreteFir  Coefficients=1/N/Ts*[1 zeros(1,N-1) -1]  InitialStates=Q0  SampleTime=Ts
  Discrete Filter : DiscreteFilter  Numerator=[0 Ts]  Denominator=[1 -1]  InitialStates=Q0  SampleTime=Ts
  y : Outport
  dy : Outport  Port=2
  wires:
  Discrete FIR Filter1/1 -> Discrete Filter/1, dy/1
  x/1 -> Discrete FIR Filter1/1
  Discrete Filter/1 -> y/1

== system TrajectoryGenerator2DOF_freq/Trajectory Generator/M23 ==
  x : Inport
  Discrete FIR Filter1 : DiscreteFir  Coefficients=1/N/Ts*[1 zeros(1,N-1) -1]  InitialStates=Q0  SampleTime=Ts
  Discrete Filter : DiscreteFilter  Numerator=[0 Ts]  Denominator=[1 -1]  InitialStates=Q0  SampleTime=Ts
  y : Outport
  dy : Outport  Port=2
  wires:
  Discrete FIR Filter1/1 -> Discrete Filter/1, dy/1
  x/1 -> Discrete FIR Filter1/1
  Discrete Filter/1 -> y/1

== system TrajectoryGenerator2DOF_freq/Trajectory Generator/M24 ==
  x : Inport
  Discrete FIR Filter1 : DiscreteFir  Coefficients=1/N/Ts*[1 zeros(1,N-1) -1]  InitialStates=Q0  SampleTime=Ts
  Discrete Filter : DiscreteFilter  Numerator=[0 Ts]  Denominator=[1 -1]  InitialStates=Q0  SampleTime=Ts
  y : Outport
  dy : Outport  Port=2
  wires:
  Discrete FIR Filter1/1 -> Discrete Filter/1, dy/1
  x/1 -> Discrete FIR Filter1/1
  Discrete Filter/1 -> y/1

== system TrajectoryGenerator2DOF_freq/Trajectory Generator/M33 ==
  x : Inport
  Discrete FIR Filter1 : DiscreteFir  Coefficients=1/N/Ts*[1 zeros(1,N-1) -1]  InitialStates=Q0  SampleTime=Ts
  Discrete Filter : DiscreteFilter  Numerator=[0 Ts]  Denominator=[1 -1]  InitialStates=Q0  SampleTime=Ts
  y : Outport
  dy : Outport  Port=2
  wires:
  Discrete FIR Filter1/1 -> Discrete Filter/1, dy/1
  x/1 -> Discrete FIR Filter1/1
  Discrete Filter/1 -> y/1

== system TrajectoryGenerator2DOF_freq/Trajectory Generator/M34 ==
  x : Inport
  Discrete FIR Filter1 : DiscreteFir  Coefficients=1/N/Ts*[1 zeros(1,N-1) -1]  InitialStates=Q0  SampleTime=Ts
  Discrete Filter : DiscreteFilter  Numerator=[0 Ts]  Denominator=[1 -1]  InitialStates=Q0  SampleTime=Ts
  y : Outport
  dy : Outport  Port=2
  wires:
  Discrete FIR Filter1/1 -> Discrete Filter/1, dy/1
  x/1 -> Discrete FIR Filter1/1
  Discrete Filter/1 -> y/1

== system TrajectoryGenerator2DOF_freq/Trajectory Generator/M44 ==
  x : Inport
  Discrete FIR Filter1 : DiscreteFir  Coefficients=1/N/Ts*[1 zeros(1,N-1) -1]  InitialStates=Q0  SampleTime=Ts
  Discrete Filter : DiscreteFilter  Numerator=[0 Ts]  Denominator=[1 -1]  InitialStates=Q0  SampleTime=Ts
  y : Outport
  dy : Outport  Port=2
  wires:
  Discrete FIR Filter1/1 -> Discrete Filter/1, dy/1
  x/1 -> Discrete FIR Filter1/1
  Discrete Filter/1 -> y/1

== system TrajectoryGenerator2DOF_freq/Trajectory Generator1/M11 ==
  x : Inport
  Discrete FIR Filter1 : DiscreteFir  Coefficients=1/N/Ts*[1 zeros(1,N-1) -1]  InitialStates=Q0  SampleTime=Ts
  Discrete Filter : DiscreteFilter  Numerator=[0 Ts]  Denominator=[1 -1]  InitialStates=Q0  SampleTime=Ts
  y : Outport
  dy : Outport  Port=2
  wires:
  Discrete FIR Filter1/1 -> Discrete Filter/1, dy/1
  x/1 -> Discrete FIR Filter1/1
  Discrete Filter/1 -> y/1

== system TrajectoryGenerator2DOF_freq/Trajectory Generator1/M12 ==
  x : Inport
  Discrete FIR Filter1 : DiscreteFir  Coefficients=1/N/Ts*[1 zeros(1,N-1) -1]  InitialStates=Q0  SampleTime=Ts
  Discrete Filter : DiscreteFilter  Numerator=[0 Ts]  Denominator=[1 -1]  InitialStates=Q0  SampleTime=Ts
  y : Outport
  dy : Outport  Port=2
  wires:
  Discrete FIR Filter1/1 -> Discrete Filter/1, dy/1
  x/1 -> Discrete FIR Filter1/1
  Discrete Filter/1 -> y/1

== system TrajectoryGenerator2DOF_freq/Trajectory Generator1/M13 ==
  x : Inport
  Discrete FIR Filter1 : DiscreteFir  Coefficients=1/N/Ts*[1 zeros(1,N-1) -1]  InitialStates=Q0  SampleTime=Ts
  Discrete Filter : DiscreteFilter  Numerator=[0 Ts]  Denominator=[1 -1]  InitialStates=Q0  SampleTime=Ts
  y : Outport
  dy : Outport  Port=2
  wires:
  Discrete FIR Filter1/1 -> Discrete Filter/1, dy/1
  x/1 -> Discrete FIR Filter1/1
  Discrete Filter/1 -> y/1

== system TrajectoryGenerator2DOF_freq/Trajectory Generator1/M14 ==
  x : Inport
  Discrete FIR Filter1 : DiscreteFir  Coefficients=1/N/Ts*[1 zeros(1,N-1) -1]  InitialStates=Q0  SampleTime=Ts
  Discrete Filter : DiscreteFilter  Numerator=[0 Ts]  Denominator=[1 -1]  InitialStates=Q0  SampleTime=Ts
  y : Outport
  dy : Outport  Port=2
  wires:
  Discrete FIR Filter1/1 -> Discrete Filter/1, dy/1
  x/1 -> Discrete FIR Filter1/1
  Discrete Filter/1 -> y/1

== system TrajectoryGenerator2DOF_freq/Trajectory Generator1/M22 ==
  x : Inport
  Discrete FIR Filter1 : DiscreteFir  Coefficients=1/N/Ts*[1 zeros(1,N-1) -1]  InitialStates=Q0  SampleTime=Ts
  Discrete Filter : DiscreteFilter  Numerator=[0 Ts]  Denominator=[1 -1]  InitialStates=Q0  SampleTime=Ts
  y : Outport
  dy : Outport  Port=2
  wires:
  Discrete FIR Filter1/1 -> Discrete Filter/1, dy/1
  x/1 -> Discrete FIR Filter1/1
  Discrete Filter/1 -> y/1

== system TrajectoryGenerator2DOF_freq/Trajectory Generator1/M23 ==
  x : Inport
  Discrete FIR Filter1 : DiscreteFir  Coefficients=1/N/Ts*[1 zeros(1,N-1) -1]  InitialStates=Q0  SampleTime=Ts
  Discrete Filter : DiscreteFilter  Numerator=[0 Ts]  Denominator=[1 -1]  InitialStates=Q0  SampleTime=Ts
  y : Outport
  dy : Outport  Port=2
  wires:
  Discrete FIR Filter1/1 -> Discrete Filter/1, dy/1
  x/1 -> Discrete FIR Filter1/1
  Discrete Filter/1 -> y/1

== system TrajectoryGenerator2DOF_freq/Trajectory Generator1/M24 ==
  x : Inport
  Discrete FIR Filter1 : DiscreteFir  Coefficients=1/N/Ts*[1 zeros(1,N-1) -1]  InitialStates=Q0  SampleTime=Ts
  Discrete Filter : DiscreteFilter  Numerator=[0 Ts]  Denominator=[1 -1]  InitialStates=Q0  SampleTime=Ts
  y : Outport
  dy : Outport  Port=2
  wires:
  Discrete FIR Filter1/1 -> Discrete Filter/1, dy/1
  x/1 -> Discrete FIR Filter1/1
  Discrete Filter/1 -> y/1

== system TrajectoryGenerator2DOF_freq/Trajectory Generator1/M33 ==
  x : Inport
  Discrete FIR Filter1 : DiscreteFir  Coefficients=1/N/Ts*[1 zeros(1,N-1) -1]  InitialStates=Q0  SampleTime=Ts
  Discrete Filter : DiscreteFilter  Numerator=[0 Ts]  Denominator=[1 -1]  InitialStates=Q0  SampleTime=Ts
  y : Outport
  dy : Outport  Port=2
  wires:
  Discrete FIR Filter1/1 -> Discrete Filter/1, dy/1
  x/1 -> Discrete FIR Filter1/1
  Discrete Filter/1 -> y/1

== system TrajectoryGenerator2DOF_freq/Trajectory Generator1/M34 ==
  x : Inport
  Discrete FIR Filter1 : DiscreteFir  Coefficients=1/N/Ts*[1 zeros(1,N-1) -1]  InitialStates=Q0  SampleTime=Ts
  Discrete Filter : DiscreteFilter  Numerator=[0 Ts]  Denominator=[1 -1]  InitialStates=Q0  SampleTime=Ts
  y : Outport
  dy : Outport  Port=2
  wires:
  Discrete FIR Filter1/1 -> Discrete Filter/1, dy/1
  x/1 -> Discrete FIR Filter1/1
  Discrete Filter/1 -> y/1

== system TrajectoryGenerator2DOF_freq/Trajectory Generator1/M44 ==
  x : Inport
  Discrete FIR Filter1 : DiscreteFir  Coefficients=1/N/Ts*[1 zeros(1,N-1) -1]  InitialStates=Q0  SampleTime=Ts
  Discrete Filter : DiscreteFilter  Numerator=[0 Ts]  Denominator=[1 -1]  InitialStates=Q0  SampleTime=Ts
  y : Outport
  dy : Outport  Port=2
  wires:
  Discrete FIR Filter1/1 -> Discrete Filter/1, dy/1
  x/1 -> Discrete FIR Filter1/1
  Discrete Filter/1 -> y/1

== system TrajectoryGenerator2DOF_freq/Trajectory Generator2/M11 ==
  x : Inport
  Discrete FIR Filter1 : DiscreteFir  Coefficients=1/N/Ts*[1 zeros(1,N-1) -1]  InitialStates=Q0  SampleTime=Ts
  Discrete Filter : DiscreteFilter  Numerator=[0 Ts]  Denominator=[1 -1]  InitialStates=Q0  SampleTime=Ts
  y : Outport
  dy : Outport  Port=2
  wires:
  Discrete FIR Filter1/1 -> Discrete Filter/1, dy/1
  x/1 -> Discrete FIR Filter1/1
  Discrete Filter/1 -> y/1

== system TrajectoryGenerator2DOF_freq/Trajectory Generator2/M12 ==
  x : Inport
  Discrete FIR Filter1 : DiscreteFir  Coefficients=1/N/Ts*[1 zeros(1,N-1) -1]  InitialStates=Q0  SampleTime=Ts
  Discrete Filter : DiscreteFilter  Numerator=[0 Ts]  Denominator=[1 -1]  InitialStates=Q0  SampleTime=Ts
  y : Outport
  dy : Outport  Port=2
  wires:
  Discrete FIR Filter1/1 -> Discrete Filter/1, dy/1
  x/1 -> Discrete FIR Filter1/1
  Discrete Filter/1 -> y/1

== system TrajectoryGenerator2DOF_freq/Trajectory Generator2/M13 ==
  x : Inport
  Discrete FIR Filter1 : DiscreteFir  Coefficients=1/N/Ts*[1 zeros(1,N-1) -1]  InitialStates=Q0  SampleTime=Ts
  Discrete Filter : DiscreteFilter  Numerator=[0 Ts]  Denominator=[1 -1]  InitialStates=Q0  SampleTime=Ts
  y : Outport
  dy : Outport  Port=2
  wires:
  Discrete FIR Filter1/1 -> Discrete Filter/1, dy/1
  x/1 -> Discrete FIR Filter1/1
  Discrete Filter/1 -> y/1

== system TrajectoryGenerator2DOF_freq/Trajectory Generator2/M14 ==
  x : Inport
  Discrete FIR Filter1 : DiscreteFir  Coefficients=1/N/Ts*[1 zeros(1,N-1) -1]  InitialStates=Q0  SampleTime=Ts
  Discrete Filter : DiscreteFilter  Numerator=[0 Ts]  Denominator=[1 -1]  InitialStates=Q0  SampleTime=Ts
  y : Outport
  dy : Outport  Port=2
  wires:
  Discrete FIR Filter1/1 -> Discrete Filter/1, dy/1
  x/1 -> Discrete FIR Filter1/1
  Discrete Filter/1 -> y/1

== system TrajectoryGenerator2DOF_freq/Trajectory Generator2/M22 ==
  x : Inport
  Discrete FIR Filter1 : DiscreteFir  Coefficients=1/N/Ts*[1 zeros(1,N-1) -1]  InitialStates=Q0  SampleTime=Ts
  Discrete Filter : DiscreteFilter  Numerator=[0 Ts]  Denominator=[1 -1]  InitialStates=Q0  SampleTime=Ts
  y : Outport
  dy : Outport  Port=2
  wires:
  Discrete FIR Filter1/1 -> Discrete Filter/1, dy/1
  x/1 -> Discrete FIR Filter1/1
  Discrete Filter/1 -> y/1

== system TrajectoryGenerator2DOF_freq/Trajectory Generator2/M23 ==
  x : Inport
  Discrete FIR Filter1 : DiscreteFir  Coefficients=1/N/Ts*[1 zeros(1,N-1) -1]  InitialStates=Q0  SampleTime=Ts
  Discrete Filter : DiscreteFilter  Numerator=[0 Ts]  Denominator=[1 -1]  InitialStates=Q0  SampleTime=Ts
  y : Outport
  dy : Outport  Port=2
  wires:
  Discrete FIR Filter1/1 -> Discrete Filter/1, dy/1
  x/1 -> Discrete FIR Filter1/1
  Discrete Filter/1 -> y/1

== system TrajectoryGenerator2DOF_freq/Trajectory Generator2/M24 ==
  x : Inport
  Discrete FIR Filter1 : DiscreteFir  Coefficients=1/N/Ts*[1 zeros(1,N-1) -1]  InitialStates=Q0  SampleTime=Ts
  Discrete Filter : DiscreteFilter  Numerator=[0 Ts]  Denominator=[1 -1]  InitialStates=Q0  SampleTime=Ts
  y : Outport
  dy : Outport  Port=2
  wires:
  Discrete FIR Filter1/1 -> Discrete Filter/1, dy/1
  x/1 -> Discrete FIR Filter1/1
  Discrete Filter/1 -> y/1

== system TrajectoryGenerator2DOF_freq/Trajectory Generator2/M33 ==
  x : Inport
  Discrete FIR Filter1 : DiscreteFir  Coefficients=1/N/Ts*[1 zeros(1,N-1) -1]  InitialStates=Q0  SampleTime=Ts
  Discrete Filter : DiscreteFilter  Numerator=[0 Ts]  Denominator=[1 -1]  InitialStates=Q0  SampleTime=Ts
  y : Outport
  dy : Outport  Port=2
  wires:
  Discrete FIR Filter1/1 -> Discrete Filter/1, dy/1
  x/1 -> Discrete FIR Filter1/1
  Discrete Filter/1 -> y/1

== system TrajectoryGenerator2DOF_freq/Trajectory Generator2/M34 ==
  x : Inport
  Discrete FIR Filter1 : DiscreteFir  Coefficients=1/N/Ts*[1 zeros(1,N-1) -1]  InitialStates=Q0  SampleTime=Ts
  Discrete Filter : DiscreteFilter  Numerator=[0 Ts]  Denominator=[1 -1]  InitialStates=Q0  SampleTime=Ts
  y : Outport
  dy : Outport  Port=2
  wires:
  Discrete FIR Filter1/1 -> Discrete Filter/1, dy/1
  x/1 -> Discrete FIR Filter1/1
  Discrete Filter/1 -> y/1

== system TrajectoryGenerator2DOF_freq/Trajectory Generator2/M44 ==
  x : Inport
  Discrete FIR Filter1 : DiscreteFir  Coefficients=1/N/Ts*[1 zeros(1,N-1) -1]  InitialStates=Q0  SampleTime=Ts
  Discrete Filter : DiscreteFilter  Numerator=[0 Ts]  Denominator=[1 -1]  InitialStates=Q0  SampleTime=Ts
  y : Outport
  dy : Outport  Port=2
  wires:
  Discrete FIR Filter1/1 -> Discrete Filter/1, dy/1
  x/1 -> Discrete FIR Filter1/1
  Discrete Filter/1 -> y/1

== system TrajectoryGenerator2DOF_freq/Trajectory Generator3/M11 ==
  x : Inport
  Discrete FIR Filter1 : DiscreteFir  Coefficients=1/N/Ts*[1 zeros(1,N-1) -1]  InitialStates=Q0  SampleTime=Ts
  Discrete Filter : DiscreteFilter  Numerator=[0 Ts]  Denominator=[1 -1]  InitialStates=Q0  SampleTime=Ts
  y : Outport
  dy : Outport  Port=2
  wires:
  Discrete FIR Filter1/1 -> Discrete Filter/1, dy/1
  x/1 -> Discrete FIR Filter1/1
  Discrete Filter/1 -> y/1

== system TrajectoryGenerator2DOF_freq/Trajectory Generator3/M12 ==
  x : Inport
  Discrete FIR Filter1 : DiscreteFir  Coefficients=1/N/Ts*[1 zeros(1,N-1) -1]  InitialStates=Q0  SampleTime=Ts
  Discrete Filter : DiscreteFilter  Numerator=[0 Ts]  Denominator=[1 -1]  InitialStates=Q0  SampleTime=Ts
  y : Outport
  dy : Outport  Port=2
  wires:
  Discrete FIR Filter1/1 -> Discrete Filter/1, dy/1
  x/1 -> Discrete FIR Filter1/1
  Discrete Filter/1 -> y/1

== system TrajectoryGenerator2DOF_freq/Trajectory Generator3/M13 ==
  x : Inport
  Discrete FIR Filter1 : DiscreteFir  Coefficients=1/N/Ts*[1 zeros(1,N-1) -1]  InitialStates=Q0  SampleTime=Ts
  Discrete Filter : DiscreteFilter  Numerator=[0 Ts]  Denominator=[1 -1]  InitialStates=Q0  SampleTime=Ts
  y : Outport
  dy : Outport  Port=2
  wires:
  Discrete FIR Filter1/1 -> Discrete Filter/1, dy/1
  x/1 -> Discrete FIR Filter1/1
  Discrete Filter/1 -> y/1

== system TrajectoryGenerator2DOF_freq/Trajectory Generator3/M14 ==
  x : Inport
  Discrete FIR Filter1 : DiscreteFir  Coefficients=1/N/Ts*[1 zeros(1,N-1) -1]  InitialStates=Q0  SampleTime=Ts
  Discrete Filter : DiscreteFilter  Numerator=[0 Ts]  Denominator=[1 -1]  InitialStates=Q0  SampleTime=Ts
  y : Outport
  dy : Outport  Port=2
  wires:
  Discrete FIR Filter1/1 -> Discrete Filter/1, dy/1
  x/1 -> Discrete FIR Filter1/1
  Discrete Filter/1 -> y/1

== system TrajectoryGenerator2DOF_freq/Trajectory Generator3/M22 ==
  x : Inport
  Discrete FIR Filter1 : DiscreteFir  Coefficients=1/N/Ts*[1 zeros(1,N-1) -1]  InitialStates=Q0  SampleTime=Ts
  Discrete Filter : DiscreteFilter  Numerator=[0 Ts]  Denominator=[1 -1]  InitialStates=Q0  SampleTime=Ts
  y : Outport
  dy : Outport  Port=2
  wires:
  Discrete FIR Filter1/1 -> Discrete Filter/1, dy/1
  x/1 -> Discrete FIR Filter1/1
  Discrete Filter/1 -> y/1

== system TrajectoryGenerator2DOF_freq/Trajectory Generator3/M23 ==
  x : Inport
  Discrete FIR Filter1 : DiscreteFir  Coefficients=1/N/Ts*[1 zeros(1,N-1) -1]  InitialStates=Q0  SampleTime=Ts
  Discrete Filter : DiscreteFilter  Numerator=[0 Ts]  Denominator=[1 -1]  InitialStates=Q0  SampleTime=Ts
  y : Outport
  dy : Outport  Port=2
  wires:
  Discrete FIR Filter1/1 -> Discrete Filter/1, dy/1
  x/1 -> Discrete FIR Filter1/1
  Discrete Filter/1 -> y/1

== system TrajectoryGenerator2DOF_freq/Trajectory Generator3/M24 ==
  x : Inport
  Discrete FIR Filter1 : DiscreteFir  Coefficients=1/N/Ts*[1 zeros(1,N-1) -1]  InitialStates=Q0  SampleTime=Ts
  Discrete Filter : DiscreteFilter  Numerator=[0 Ts]  Denominator=[1 -1]  InitialStates=Q0  SampleTime=Ts
  y : Outport
  dy : Outport  Port=2
  wires:
  Discrete FIR Filter1/1 -> Discrete Filter/1, dy/1
  x/1 -> Discrete FIR Filter1/1
  Discrete Filter/1 -> y/1

== system TrajectoryGenerator2DOF_freq/Trajectory Generator3/M33 ==
  x : Inport
  Discrete FIR Filter1 : DiscreteFir  Coefficients=1/N/Ts*[1 zeros(1,N-1) -1]  InitialStates=Q0  SampleTime=Ts
  Discrete Filter : DiscreteFilter  Numerator=[0 Ts]  Denominator=[1 -1]  InitialStates=Q0  SampleTime=Ts
  y : Outport
  dy : Outport  Port=2
  wires:
  Discrete FIR Filter1/1 -> Discrete Filter/1, dy/1
  x/1 -> Discrete FIR Filter1/1
  Discrete Filter/1 -> y/1

== system TrajectoryGenerator2DOF_freq/Trajectory Generator3/M34 ==
  x : Inport
  Discrete FIR Filter1 : DiscreteFir  Coefficients=1/N/Ts*[1 zeros(1,N-1) -1]  InitialStates=Q0  SampleTime=Ts
  Discrete Filter : DiscreteFilter  Numerator=[0 Ts]  Denominator=[1 -1]  InitialStates=Q0  SampleTime=Ts
  y : Outport
  dy : Outport  Port=2
  wires:
  Discrete FIR Filter1/1 -> Discrete Filter/1, dy/1
  x/1 -> Discrete FIR Filter1/1
  Discrete Filter/1 -> y/1

== system TrajectoryGenerator2DOF_freq/Trajectory Generator3/M44 ==
  x : Inport
  Discrete FIR Filter1 : DiscreteFir  Coefficients=1/N/Ts*[1 zeros(1,N-1) -1]  InitialStates=Q0  SampleTime=Ts
  Discrete Filter : DiscreteFilter  Numerator=[0 Ts]  Denominator=[1 -1]  InitialStates=Q0  SampleTime=Ts
  y : Outport
  dy : Outport  Port=2
  wires:
  Discrete FIR Filter1/1 -> Discrete Filter/1, dy/1
  x/1 -> Discrete FIR Filter1/1
  Discrete Filter/1 -> y/1

== system TrajectoryGenerator2DOF_freq/Trajectory Generator4/M11 ==
  x : Inport
  Discrete FIR Filter1 : DiscreteFir  Coefficients=1/N/Ts*[1 zeros(1,N-1) -1]  InitialStates=Q0  SampleTime=Ts
  Discrete Filter : DiscreteFilter  Numerator=[0 Ts]  Denominator=[1 -1]  InitialStates=Q0  SampleTime=Ts
  y : Outport
  dy : Outport  Port=2
  wires:
  Discrete FIR Filter1/1 -> Discrete Filter/1, dy/1
  x/1 -> Discrete FIR Filter1/1
  Discrete Filter/1 -> y/1
